simulink model "Simulation"  (R2020b)
settings: Solver=VariableStepAuto  StartTime=0.0  StopTime=0.5  MaxStep=1e-6  RelTol=1e-3
values from neighbouring files (symbols this model uses):
  K = 4.7    [Parametres.m]
  Kd = ((ALPHAA+(2*DD))*W00)/0.654    (= 229.357798165)    [Parametres.m]
  Ki = 28575.5    [Parametres.m]
  Kii = (ALPHAA*(W00^3))/0.654    (= 191131.498471)    [Parametres.m]
  Kp = 33.64    [Parametres.m]
  Kpp = (((1+(2*ALPHAA*DD))*(W00^2))+872)/0.654    (= 12801.2232416)    [Parametres.m]
  T1 = 0.075    [Parametres.m]
  Tlaser = 1/(2*pi*2500)    (= 6.36619772368e-05)    [Parametres.m]
  Ts = 100e-6    (= 0.0001)    [Parametres.m]
  Tt = 0.0005    [Parametres.m]
  Tt2 = ((Kii/Kpp)*(Kd/Kpp))^0.5    (= 0.517215362986)    [Parametres.m]
libraries: simulink x2, cstblocks x1, simulink_extras x1
settings Model: Creator=TAHABDESSALEM MERAD  LastModifiedBy=TAHABDESSALEM MERAD

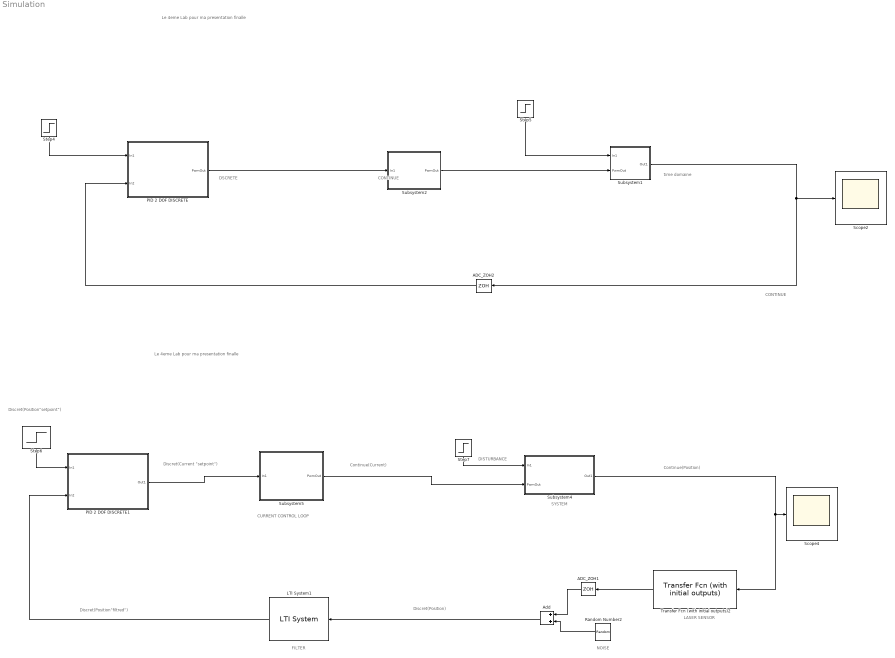
== system Simulation ==
  note: CURRENT CONTROL LOOP
  note: LASER SENSOR
  note: NOISE
  note: DISTURBANCE
  note: SYSTEM
  note: FILTER
  note: CONTINUE
  note: CONTINUE
  note: time domaine
  note: Continue(Position)
  note: DSCRETE
  note: Continue(Current)
  note: Discret(Position"filtred")
  note: Discret(Position)
  note: Discret(Current "setpoint")
  note: Discret(Position"setpoint")
  note: Le 4eme Lab pour ma presentation finalle
  note: Le 4eme Lab pour ma presentation finalle
  " PID 2 DOF DISCRETE" : Subsystem
  " PID 2 DOF DISCRETE1" : Subsystem
  ADC_ZOH1 : ZeroOrderHold  SampleTime=100e-6
  ADC_ZOH2 : ZeroOrderHold  SampleTime=100e-6
  Add : Sum
  LTI System1 : cstblocks/LTI System  sys=FLTDSC  IC=[]
  Random Number2 : RandomNumber  Variance=(0.00025)^2  SampleTime=0.0001
  Scope2 : Scope
  Scope4 : Scope
  Step4 : Step  Time=0  After=0.003  SampleTime=100e-6
  Step5 : Step  Time=0.2  After=10  SampleTime=100e-6
  Step6 : Step  Time=0  After=0.003  SampleTime=100e-6
  Step7 : Step  Time=0.2  After=10  SampleTime=100e-6
  Subsystem1 : Subsystem
  Subsystem2 : Subsystem
  Subsystem4 : Subsystem
  Subsystem5 : Subsystem
  Transfer Fcn (with initial outputs)2 : simulink_extras/Additional Linear/Transfer Fcn (with initial outputs)  N=[1]  D="[Tlaser  1]"  Y0=0  U0=0
  wires:
  ADC_ZOH2/1 -> " PID 2 DOF DISCRETE"/2(In2)
  Step5/1 -> Subsystem1/1(In1)
  " PID 2 DOF DISCRETE"/1(PwmOut) -> Subsystem2/1(In1)
  Step6/1 -> " PID 2 DOF DISCRETE1"/1(In1)
  Step4/1 -> " PID 2 DOF DISCRETE"/1(In1)
  Step7/1 -> Subsystem4/1(In1)
  " PID 2 DOF DISCRETE1"/1(Out1) -> Subsystem5/1(In1)
  Subsystem1/1(Out1) -> ADC_ZOH2/1, Scope2/1
  Subsystem5/1(PwmOut) -> Subsystem4/2(PwmOut)
  Transfer Fcn (with initial outputs)2/1 -> ADC_ZOH1/1
  Subsystem4/1(Out1) -> Transfer Fcn (with initial outputs)2/1, Scope4/1
  ADC_ZOH1/1 -> Add/1
  Random Number2/1 -> Add/2
  Add/1 -> LTI System1/1
  LTI System1/1 -> " PID 2 DOF DISCRETE1"/2(In2)
  Subsystem2/1(PwmOut) -> Subsystem1/2(PwmOut)

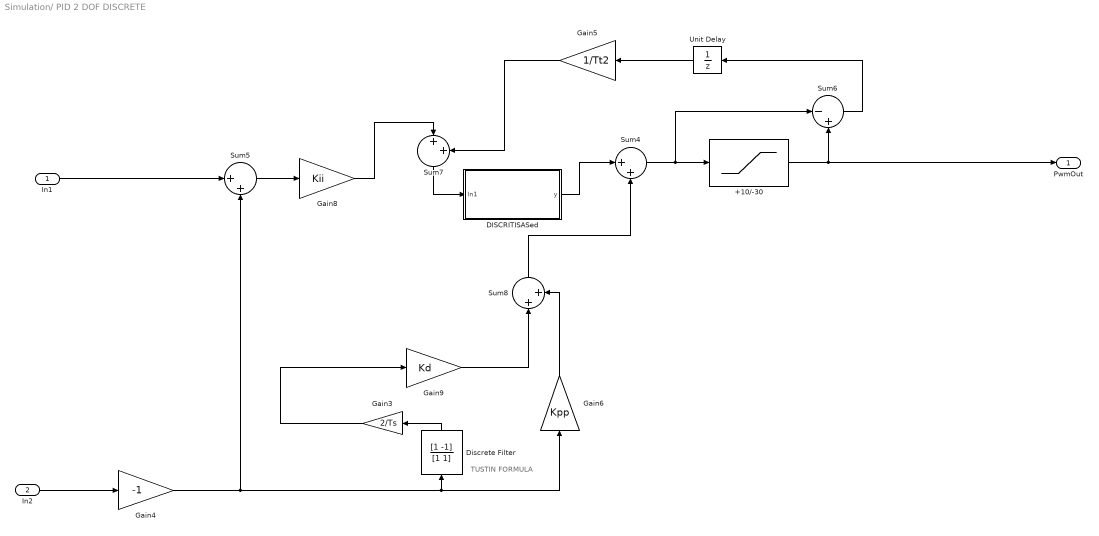
== system Simulation/ PID 2 DOF DISCRETE ==
  note: TUSTIN FORMULA
  In1 : Inport
  In2 : Inport  Port=2
  +10/-30 : Saturate  UpperLimit=+10  LowerLimit=-30
  DISCRITISASed : Subsystem
  Discrete Filter : DiscreteFilter  Numerator=[1 -1]  Denominator=[1 1]  SampleTime=Ts
  Gain3 : Gain  Gain=2/Ts
  Gain4 : Gain  Gain=-1
  Gain5 : Gain  Gain=1/Tt2
  Gain6 : Gain  Gain=Kpp
  Gain8 : Gain  Gain=Kii
  Gain9 : Gain  Gain=Kd
  Sum{4..5,7..8} (4 alike) : Sum  Inputs=|++
  Sum6 : Sum  Inputs=|-+
  Unit Delay : UnitDelay  SampleTime=-1  HasFrameUpgradeWarning=on
  PwmOut : Outport
  wires:
  In1/1 -> Sum5/1
  Sum4/1 -> Sum6/1, +10/-30/1
  DISCRITISASed/1(y) -> Sum4/1
  Gain8/1 -> Sum7/1
  Sum7/1 -> DISCRITISASed/1(In1)
  Gain6/1 -> Sum8/2
  Gain3/1 -> Gain9/1
  Gain9/1 -> Sum8/1
  Sum8/1 -> Sum4/2
  Sum5/1 -> Gain8/1
  Gain5/1 -> Sum7/2
  +10/-30/1 -> Sum6/2, PwmOut/1
  In2/1 -> Gain4/1
  Gain4/1 -> Sum5/2, Gain6/1, Discrete Filter/1
  Unit Delay/1 -> Gain5/1
  Sum6/1 -> Unit Delay/1
  Discrete Filter/1 -> Gain3/1

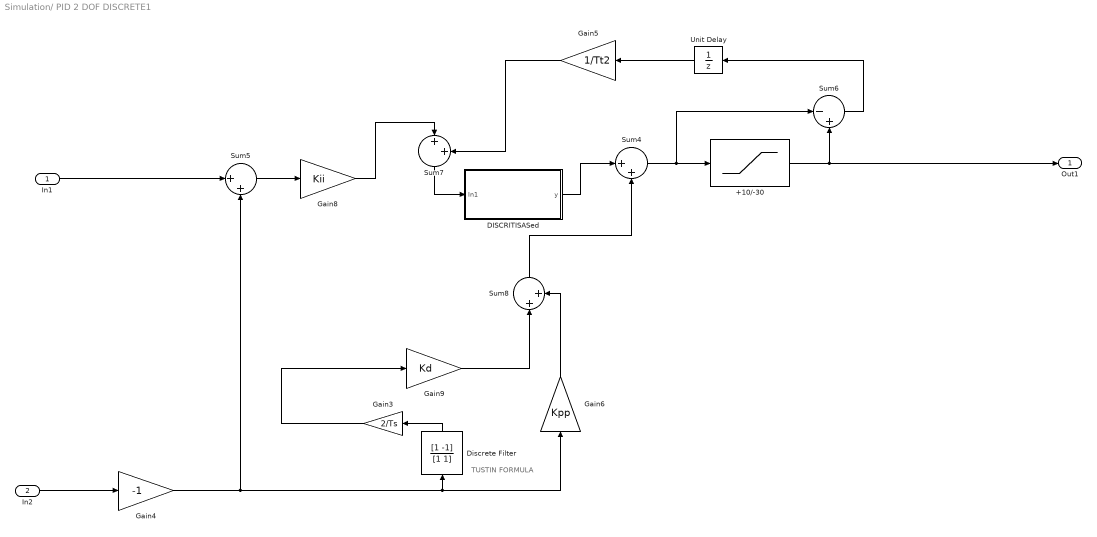
== system Simulation/ PID 2 DOF DISCRETE1 ==
  note: TUSTIN FORMULA
  In1 : Inport
  In2 : Inport  Port=2
  +10/-30 : Saturate  UpperLimit=+10  LowerLimit=-30
  DISCRITISASed : Subsystem
  Discrete Filter : DiscreteFilter  Numerator=[1 -1]  Denominator=[1 1]  SampleTime=Ts
  Gain3 : Gain  Gain=2/Ts
  Gain4 : Gain  Gain=-1
  Gain5 : Gain  Gain=1/Tt2
  Gain6 : Gain  Gain=Kpp
  Gain8 : Gain  Gain=Kii
  Gain9 : Gain  Gain=Kd
  Sum{4..5,7..8} (4 alike) : Sum  Inputs=|++
  Sum6 : Sum  Inputs=|-+
  Unit Delay : UnitDelay  SampleTime=-1  HasFrameUpgradeWarning=on
  Out1 : Outport
  wires:
  Discrete Filter/1 -> Gain3/1
  Sum6/1 -> Unit Delay/1
  Unit Delay/1 -> Gain5/1
  Gain4/1 -> Discrete Filter/1, Gain6/1, Sum5/2
  In2/1 -> Gain4/1
  +10/-30/1 -> Out1/1, Sum6/2
  Gain5/1 -> Sum7/2
  Sum5/1 -> Gain8/1
  Sum8/1 -> Sum4/2
  Gain9/1 -> Sum8/1
  Gain3/1 -> Gain9/1
  Gain6/1 -> Sum8/2
  Sum7/1 -> DISCRITISASed/1(In1)
  Gain8/1 -> Sum7/1
  DISCRITISASed/1(y) -> Sum4/1
  Sum4/1 -> +10/-30/1, Sum6/1
  In1/1 -> Sum5/1

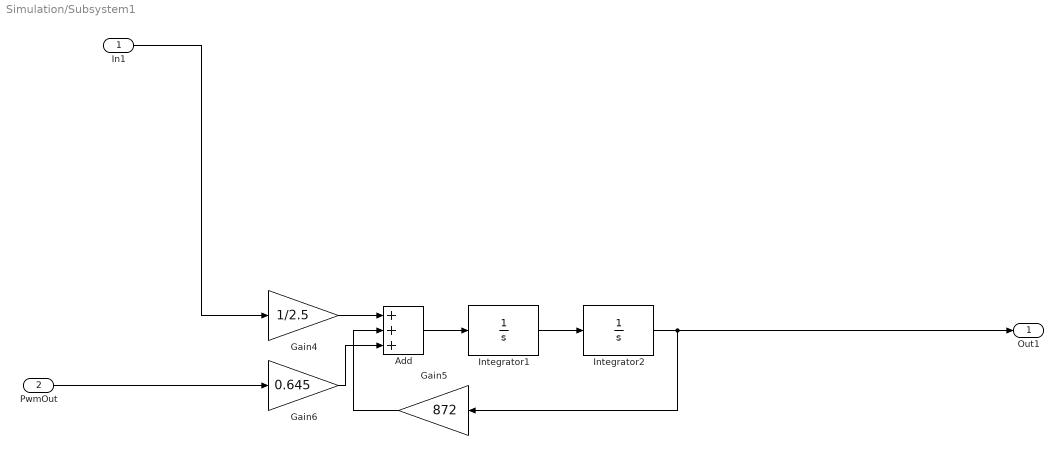
== system Simulation/Subsystem1 ==
  In1 : Inport
  PwmOut : Inport  Port=2
  Add : Sum  Inputs=+++
  Gain4 : Gain  Gain=1/2.5
  Gain5 : Gain  Gain=872
  Gain6 : Gain  Gain=0.645
  Integrator1 : Integrator
  Integrator2 : Integrator
  Out1 : Outport
  wires:
  Gain6/1 -> Add/3
  Gain4/1 -> Add/1
  Gain5/1 -> Add/2
  PwmOut/1 -> Gain6/1
  In1/1 -> Gain4/1
  Integrator1/1 -> Integrator2/1
  Integrator2/1 -> Gain5/1, Out1/1
  Add/1 -> Integrator1/1

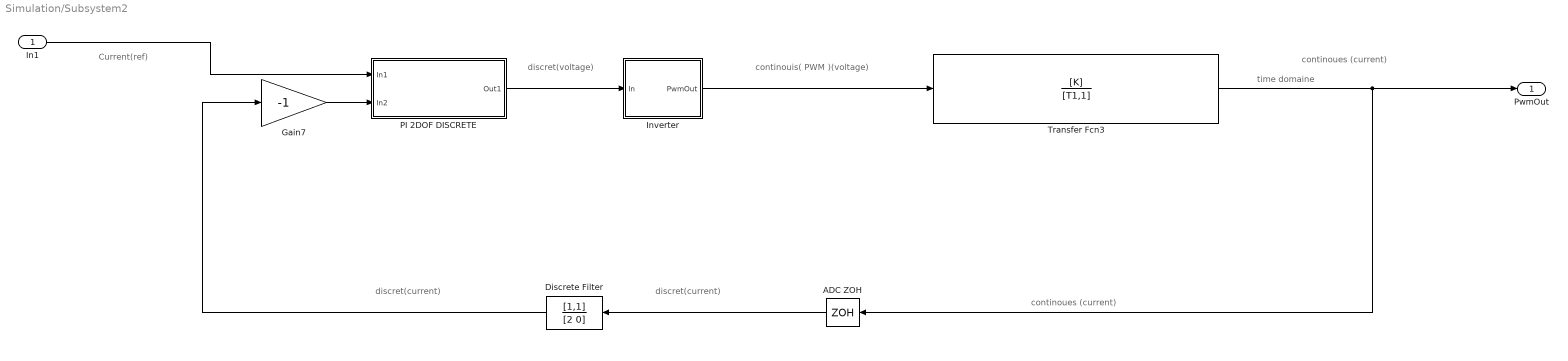
== system Simulation/Subsystem2 ==
  note: discret(current)
  note: continoues (current)
  note: continouis( PWM )(voltage)
  note: discret(voltage)
  note: Current(ref)
  note: time domaine
  note: discret(current)
  note: continoues (current)
  In1 : Inport
  ADC ZOH : ZeroOrderHold  SampleTime=100e-6
  Discrete Filter : DiscreteFilter  Numerator=[1,1]  Denominator=[2 0]
  Gain7 : Gain  Gain=-1
  Inverter : Subsystem
  PI 2DOF DISCRETE : Subsystem
  Transfer Fcn3 : TransferFcn  Numerator=[K]  Denominator=[T1,1]
  PwmOut : Outport
  wires:
  Transfer Fcn3/1 -> PwmOut/1, ADC ZOH/1
  ADC ZOH/1 -> Discrete Filter/1
  Inverter/1(PwmOut) -> Transfer Fcn3/1
  Discrete Filter/1 -> Gain7/1
  In1/1 -> PI 2DOF DISCRETE/1(In1)
  PI 2DOF DISCRETE/1(Out1) -> Inverter/1(In)
  Gain7/1 -> PI 2DOF DISCRETE/2(In2)

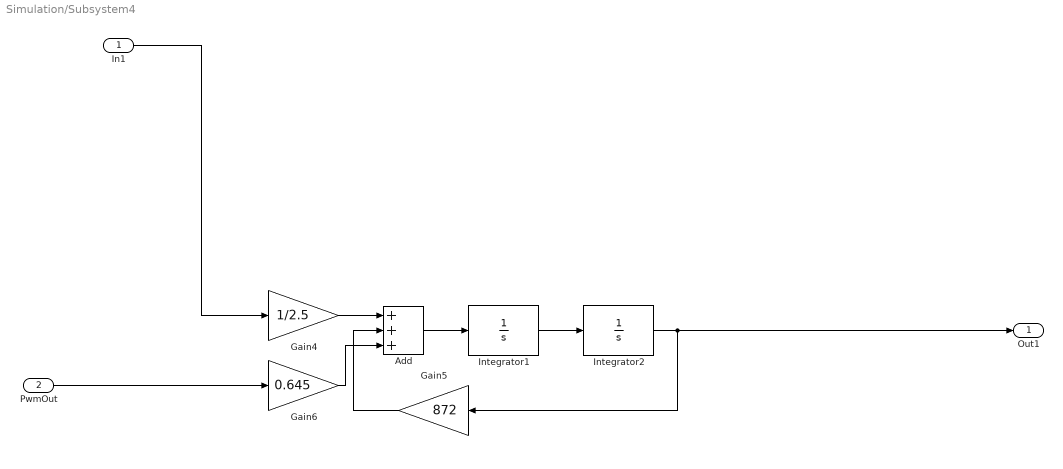
== system Simulation/Subsystem4 ==
  In1 : Inport
  PwmOut : Inport  Port=2
  Add : Sum  Inputs=+++
  Gain4 : Gain  Gain=1/2.5
  Gain5 : Gain  Gain=872
  Gain6 : Gain  Gain=0.645
  Integrator1 : Integrator
  Integrator2 : Integrator
  Out1 : Outport
  wires:
  Add/1 -> Integrator1/1
  Integrator2/1 -> Out1/1, Gain5/1
  Integrator1/1 -> Integrator2/1
  In1/1 -> Gain4/1
  PwmOut/1 -> Gain6/1
  Gain5/1 -> Add/2
  Gain4/1 -> Add/1
  Gain6/1 -> Add/3

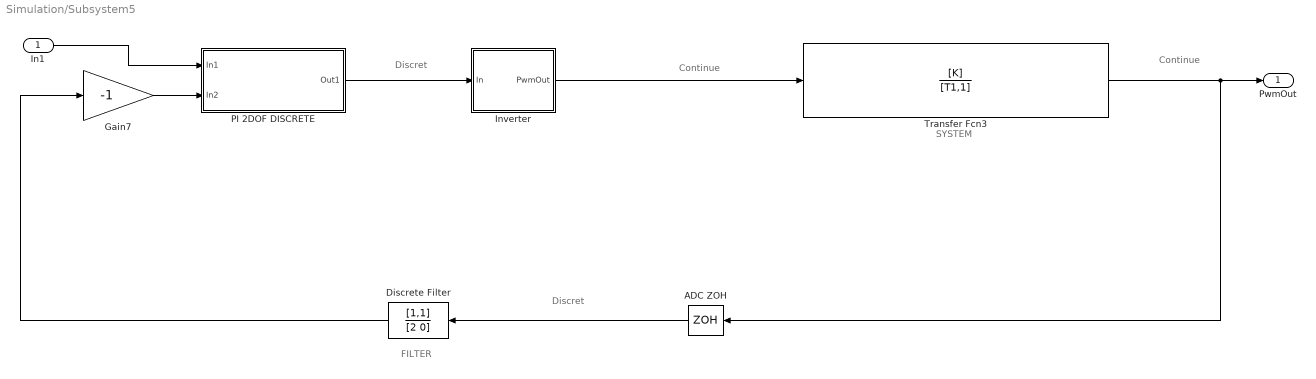
== system Simulation/Subsystem5 ==
  note: FILTER
  note: SYSTEM
  note: Discret
  note: Continue
  note: Continue
  note: Discret
  In1 : Inport
  ADC ZOH : ZeroOrderHold  SampleTime=100e-6
  Discrete Filter : DiscreteFilter  Numerator=[1,1]  Denominator=[2 0]
  Gain7 : Gain  Gain=-1
  Inverter : Subsystem
  PI 2DOF DISCRETE : Subsystem
  Transfer Fcn3 : TransferFcn  Numerator=[K]  Denominator=[T1,1]
  PwmOut : Outport
  wires:
  Transfer Fcn3/1 -> ADC ZOH/1, PwmOut/1
  ADC ZOH/1 -> Discrete Filter/1
  Inverter/1(PwmOut) -> Transfer Fcn3/1
  Discrete Filter/1 -> Gain7/1
  In1/1 -> PI 2DOF DISCRETE/1(In1)
  PI 2DOF DISCRETE/1(Out1) -> Inverter/1(In)
  Gain7/1 -> PI 2DOF DISCRETE/2(In2)

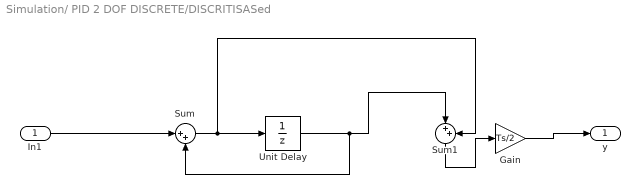
== system Simulation/ PID 2 DOF DISCRETE/DISCRITISASed ==
  In1 : Inport
  Gain : Gain  Gain=Ts/2
  Sum : Sum  Inputs=|++
  Sum1 : Sum  Inputs=|++
  Unit Delay : UnitDelay  SampleTime=-1  HasFrameUpgradeWarning=on
  y : Outport
  wires:
  In1/1 -> Sum/1
  Sum/1 -> Sum1/2, Unit Delay/1
  Unit Delay/1 -> Sum/2, Sum1/1
  Gain/1 -> y/1
  Sum1/1 -> Gain/1

== system Simulation/ PID 2 DOF DISCRETE1/DISCRITISASed ==
  In1 : Inport
  Gain : Gain  Gain=Ts/2
  Sum : Sum  Inputs=|++
  Sum1 : Sum  Inputs=|++
  Unit Delay : UnitDelay  SampleTime=-1  HasFrameUpgradeWarning=on
  y : Outport
  wires:
  Sum1/1 -> Gain/1
  Gain/1 -> y/1
  Unit Delay/1 -> Sum1/1, Sum/2
  Sum/1 -> Unit Delay/1, Sum1/2
  In1/1 -> Sum/1

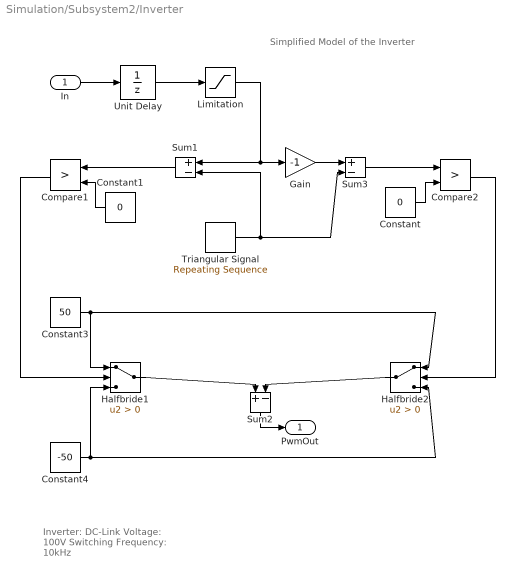
== system Simulation/Subsystem2/Inverter ==
  note: Simplified Model of the Inverter
  note: Inverter:
      | DC-Link Voltage: 100V
      | Switching Frequency: 10kHz
  In : Inport
  Compare1 : RelationalOperator  Operator=>  OutDataTypeStr=boolean  RndMeth=Nearest
  Compare2 : RelationalOperator  Operator=>  OutDataTypeStr=boolean  RndMeth=Nearest
  Constant : Constant  Value=0
  Constant1 : Constant  Value=0
  Constant3 : Constant  Value=50
  Constant4 : Constant  Value=-50
  Gain : Gain  Gain=-1
  Halfbride1 : Switch  Criteria=u2 > Threshold
  Halfbride2 : Switch  Criteria=u2 > Threshold
  Limitation : Saturate  UpperLimit=100  LowerLimit=-100
  Sum1 : Sum  Inputs=+-
  Sum2 : Sum  Inputs=+-
  Sum3 : Sum  Inputs=+-
  Triangular Signal : simulink/Sources/Repeating Sequence  rep_seq_t=[0 50e-6 100e-6]  rep_seq_y=[-100 100 -100]
  Unit Delay : UnitDelay  SampleTime=-1
  PwmOut : Outport
  wires:
  Sum3/1 -> Compare2/1
  Constant/1 -> Compare2/2
  Constant1/1 -> Compare1/2
  Sum1/1 -> Compare1/1
  Constant3/1 -> Halfbride1/1, Halfbride2/1
  Constant4/1 -> Halfbride1/3, Halfbride2/3
  Halfbride1/1 -> Sum2/1
  Halfbride2/1 -> Sum2/2
  Compare1/1 -> Halfbride1/2
  Compare2/1 -> Halfbride2/2
  Gain/1 -> Sum3/1
  Triangular Signal/1 -> Sum1/2, Sum3/2
  Limitation/1 -> Gain/1, Sum1/1
  In/1 -> Unit Delay/1
  Sum2/1 -> PwmOut/1
  Unit Delay/1 -> Limitation/1

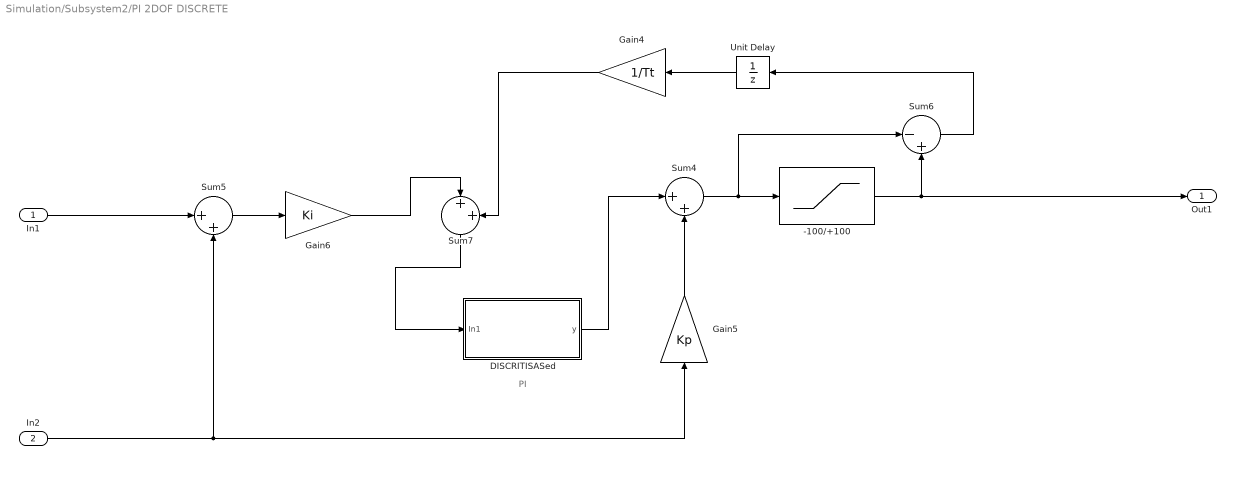
== system Simulation/Subsystem2/PI 2DOF DISCRETE ==
  note: PI
  In1 : Inport
  In2 : Inport  Port=2
  -100/+100 : Saturate  UpperLimit=60  LowerLimit=-60
  DISCRITISASed : Subsystem
  Gain4 : Gain  Gain=1/Tt
  Gain5 : Gain  Gain=Kp
  Gain6 : Gain  Gain=Ki
  Sum4 : Sum  Inputs=|++
  Sum5 : Sum  Inputs=|++
  Sum6 : Sum  Inputs=|-+
  Sum7 : Sum  Inputs=|++
  Unit Delay : UnitDelay  SampleTime=-1  HasFrameUpgradeWarning=on
  Out1 : Outport
  wires:
  In2/1 -> Gain5/1, Sum5/2
  Unit Delay/1 -> Gain4/1
  Gain4/1 -> Sum7/2
  Sum4/1 -> -100/+100/1, Sum6/1
  Sum6/1 -> Unit Delay/1
  Gain6/1 -> Sum7/1
  Sum5/1 -> Gain6/1
  Gain5/1 -> Sum4/2
  Sum7/1 -> DISCRITISASed/1(In1)
  In1/1 -> Sum5/1
  -100/+100/1 -> Out1/1, Sum6/2
  DISCRITISASed/1(y) -> Sum4/1

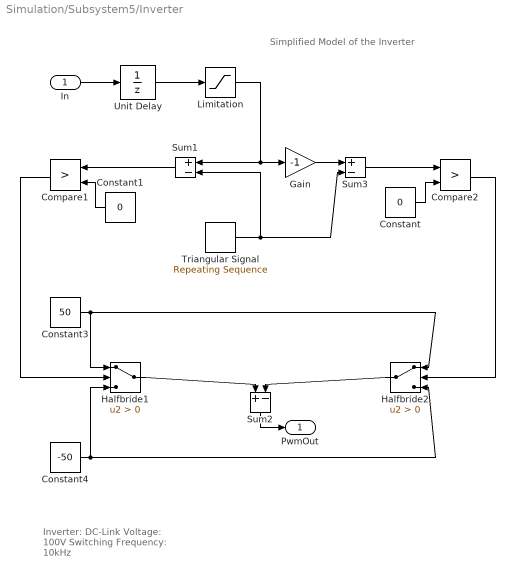
== system Simulation/Subsystem5/Inverter ==
  note: Simplified Model of the Inverter
  note: Inverter:
      | DC-Link Voltage: 100V
      | Switching Frequency: 10kHz
  In : Inport
  Compare1 : RelationalOperator  Operator=>  OutDataTypeStr=boolean  RndMeth=Nearest
  Compare2 : RelationalOperator  Operator=>  OutDataTypeStr=boolean  RndMeth=Nearest
  Constant : Constant  Value=0
  Constant1 : Constant  Value=0
  Constant3 : Constant  Value=50
  Constant4 : Constant  Value=-50
  Gain : Gain  Gain=-1
  Halfbride1 : Switch  Criteria=u2 > Threshold
  Halfbride2 : Switch  Criteria=u2 > Threshold
  Limitation : Saturate  UpperLimit=100  LowerLimit=-100
  Sum1 : Sum  Inputs=+-
  Sum2 : Sum  Inputs=+-
  Sum3 : Sum  Inputs=+-
  Triangular Signal : simulink/Sources/Repeating Sequence  rep_seq_t=[0 50e-6 100e-6]  rep_seq_y=[-100 100 -100]
  Unit Delay : UnitDelay  SampleTime=-1
  PwmOut : Outport
  wires:
  Sum3/1 -> Compare2/1
  Constant/1 -> Compare2/2
  Constant1/1 -> Compare1/2
  Sum1/1 -> Compare1/1
  Constant3/1 -> Halfbride1/1, Halfbride2/1
  Constant4/1 -> Halfbride1/3, Halfbride2/3
  Halfbride1/1 -> Sum2/1
  Halfbride2/1 -> Sum2/2
  Compare1/1 -> Halfbride1/2
  Compare2/1 -> Halfbride2/2
  Gain/1 -> Sum3/1
  Triangular Signal/1 -> Sum1/2, Sum3/2
  Limitation/1 -> Gain/1, Sum1/1
  In/1 -> Unit Delay/1
  Sum2/1 -> PwmOut/1
  Unit Delay/1 -> Limitation/1

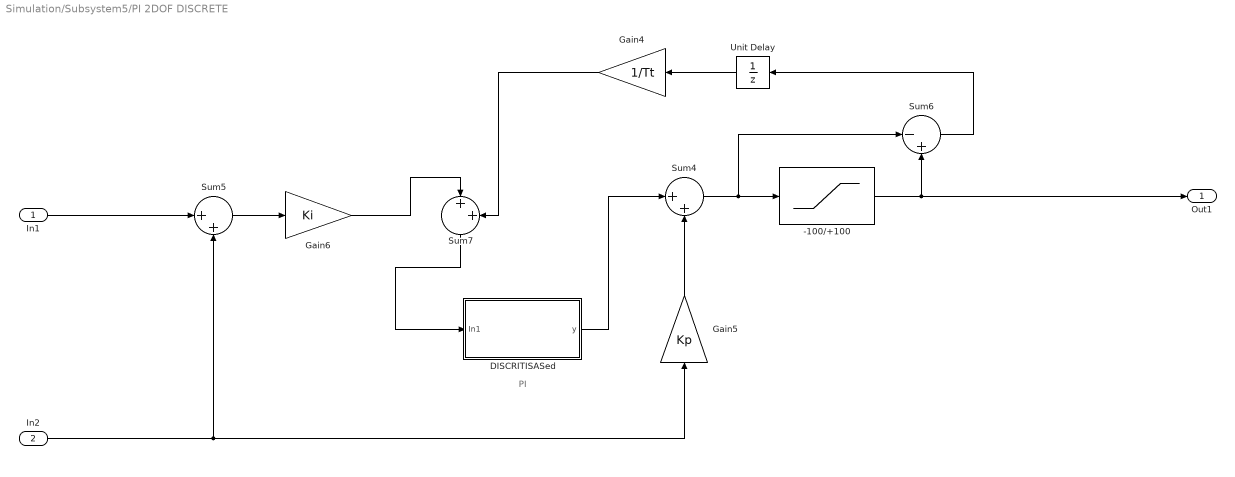
== system Simulation/Subsystem5/PI 2DOF DISCRETE ==
  note: PI
  In1 : Inport
  In2 : Inport  Port=2
  -100/+100 : Saturate  UpperLimit=60  LowerLimit=-60
  DISCRITISASed : Subsystem
  Gain4 : Gain  Gain=1/Tt
  Gain5 : Gain  Gain=Kp
  Gain6 : Gain  Gain=Ki
  Sum4 : Sum  Inputs=|++
  Sum5 : Sum  Inputs=|++
  Sum6 : Sum  Inputs=|-+
  Sum7 : Sum  Inputs=|++
  Unit Delay : UnitDelay  SampleTime=-1  HasFrameUpgradeWarning=on
  Out1 : Outport
  wires:
  In2/1 -> Gain5/1, Sum5/2
  Unit Delay/1 -> Gain4/1
  Gain4/1 -> Sum7/2
  Sum4/1 -> -100/+100/1, Sum6/1
  Sum6/1 -> Unit Delay/1
  Gain6/1 -> Sum7/1
  Sum5/1 -> Gain6/1
  Gain5/1 -> Sum4/2
  Sum7/1 -> DISCRITISASed/1(In1)
  In1/1 -> Sum5/1
  -100/+100/1 -> Out1/1, Sum6/2
  DISCRITISASed/1(y) -> Sum4/1

== system Simulation/Subsystem2/PI 2DOF DISCRETE/DISCRITISASed ==
  In1 : Inport
  Gain : Gain  Gain=Ts/2
  Sum : Sum  Inputs=|++
  Sum1 : Sum  Inputs=|++
  Unit Delay : UnitDelay  SampleTime=-1  HasFrameUpgradeWarning=on
  y : Outport
  wires:
  In1/1 -> Sum/1
  Sum/1 -> Sum1/2, Unit Delay/1
  Unit Delay/1 -> Sum/2, Sum1/1
  Gain/1 -> y/1
  Sum1/1 -> Gain/1

== system Simulation/Subsystem5/PI 2DOF DISCRETE/DISCRITISASed ==
  In1 : Inport
  Gain : Gain  Gain=Ts/2
  Sum : Sum  Inputs=|++
  Sum1 : Sum  Inputs=|++
  Unit Delay : UnitDelay  SampleTime=-1  HasFrameUpgradeWarning=on
  y : Outport
  wires:
  In1/1 -> Sum/1
  Sum/1 -> Sum1/2, Unit Delay/1
  Unit Delay/1 -> Sum/2, Sum1/1
  Gain/1 -> y/1
  Sum1/1 -> Gain/1
